simulink model "suspensionSimscapeLUT"  (R2015a)
settings: Solver=ode23t  StartTime=0.0  StopTime=10  MaxStep=1e-3  RelTol=1e-3
PreLoadFcn:
  | load carParams
  | load springData
values from neighbouring files (symbols this model uses):
  b1 = 2500    [carParams.mat]
  b2 = 15000    [carParams.mat]
libraries: fl_lib x8, nesl_utility x3, sdl_lib x1
settings Model: Creator=scastro  LastModifiedBy=chahn
settings DataIOCC: LimitDataPoints=off  OutputTimes=0:0.01:60
settings SimscapeCC: SimscapeLogType=all  SimscapeLogDataHistory=10000

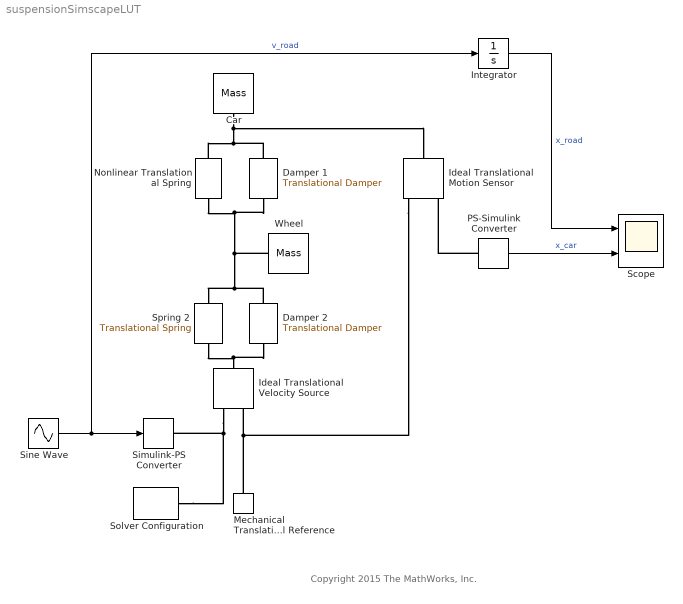
== system suspensionSimscapeLUT ==
  note: Copyright 2015 The MathWorks, Inc.
  Car : fl_lib/Mechanical/Translational Elements/Mass  mass=mCar kg  v_specify=on  v_priority=High  v=0 m/s  f_specify=off  f_priority=High  f=0 N
  Damper 1 : fl_lib/Mechanical/Translational Elements/Translational Damper  D=b1 N/(m/s)  v_specify=off  v_priority=High  v=0 m/s  f_specify=off  f_priority=High  f=0 N
  Damper 2 : fl_lib/Mechanical/Translational Elements/Translational Damper  D=b2 N/(m/s)  v_specify=off  v_priority=High  v=0 m/s  f_specify=off  f_priority=High  f=0 N
  Ideal Translational Motion Sensor : fl_lib/Mechanical/Mechanical Sensors/Ideal Translational Motion Sensor  offset=0 m
  Ideal Translational Velocity Source : fl_lib/Mechanical/Mechanical Sources/Ideal Translational Velocity Source
  Integrator : Integrator
  Mechanical Translational Reference : fl_lib/Mechanical/Translational Elements/Mechanical Translational Reference
  Nonlinear Translational Spring : sdl_lib/Couplings & Drives/Springs & Dampers/Nonlinear Translational Spring  parameterization=2  symmetry=1  coefficient_vector=[ 100 0 10 0 1 ] N/m  tension_coefficient_vector=[ 100 0 10 0 1 ] N/m  compression_coefficient_vector=[ 1000 -10 100 0 0 ] N/m  deformation_vector=x cm  force_vector=Fs N  interp_method=1  extrap_method=1  init_def=0 m
  PS-Simulink Converter : nesl_utility/PS-Simulink Converter  PhysicalDomain=network_engine_domain  SubClassName=ps_output  LeftPortType=input  RightPortType=output  PseudoPeriodic=off  Frequencies=[]  Unit=cm  AffineConversion=off
  Scope : Scope  NumInputPorts=2
      settings: TimeRange=10  YMin=-4~-0.2  YMax=4~0.2
  Simulink-PS Converter : nesl_utility/Simulink-PS Converter  PhysicalDomain=network_engine_domain  SubClassName=ps_input  LeftPortType=input  RightPortType=output  PseudoPeriodic=off  Frequencies=[]  NoiseDistribution=none  NoiseParameters=[]  Unit=cm/s  AffineConversion=off  InputFiltering=off  SimscapeFilterOrder=1  InputFilterTimeConstant=0.001  UdotUserProvided=1
  Sine Wave : Sin  Amplitude=250  Frequency=100  Phase=pi/2  SampleTime=0
  Solver Configuration : nesl_utility/Solver Configuration  PhysicalDomain=network_engine_domain  SubClassName=solver  LeftPortType=input  RightPortType=generic  Accelerate=off  Tones=[]  Harmonics=[]  SimulateNoise=off  Profile=off  UseLocalSampling=off  EnableSwitchedLinearOptims=on  FrequencyDomain=off  UseCCode=off  RelTol=0.001  AbsTol=1e-06  MinStep=1e-09  ToWorkspace=off  RevertToSquareIcSolve=off  NumHomotopyIterations=100  DoDC=off  ResidualTolerance=1e-09  UseLocalSolver=off  LocalSolverChoice=NE_BACKWARD_EULER_ADVANCER  LocalSolverSampleTime=0.001  DoFixedCost=off  MaxNonlinIter=3  MaxModeIter=2  LinearAlgebra=Sparse  DelaysMemoryBudget=1024  AutomaticFiltering=on  FilteringTimeConstant=0.001
  Spring 2 : fl_lib/Mechanical/Translational Elements/Translational Spring  spr_rate=k2 N/m  v_specify=off  v_priority=High  v=0 m/s  f_specify=off  f_priority=High  f=0 N  x_specify=on  x_priority=High  x=0 m
  Wheel : fl_lib/Mechanical/Translational Elements/Mass  mass=mWheel kg  v_specify=on  v_priority=Low  v=0 m/s  f_specify=off  f_priority=High  f=0 N
  wires:
  Sine Wave/1 -> Simulink-PS Converter/1, Integrator/1  "v_road"
  Integrator/1 -> Scope/1  "x_road"
  PS-Simulink Converter/1 -> Scope/2  "x_car"
  connections:
  Ideal Translational Velocity Source/RConn1 -- Solver Configuration/RConn1 -- Simulink-PS Converter/RConn1
  Mechanical Translational Reference/LConn1 -- Ideal Translational Motion Sensor/RConn1 -- Ideal Translational Velocity Source/RConn2
  Spring 2/RConn1 -- Damper 2/RConn1 -- Ideal Translational Velocity Source/LConn1
  Damper 1/RConn1 -- Nonlinear Translational Spring/RConn1 -- Spring 2/LConn1 -- Damper 2/LConn1 -- Wheel/LConn1
  Ideal Translational Motion Sensor/LConn1 -- Car/LConn1 -- Nonlinear Translational Spring/LConn1 -- Damper 1/LConn1
  PS-Simulink Converter/LConn1 -- Ideal Translational Motion Sensor/RConn3
